simulink model "Sliders_mdl"  (R2018b)
settings: Solver=VariableStepAuto  StartTime=0.0  StopTime=10  MaxStep=0.01  RelTol=1e-3  EnableMultiTasking=on
libraries: lpvlibrary x2, cstblocks x1, simulink x1
settings Model: Creator=Fernando  LastModifiedBy=ferna
settings OptimizationCC: LifeSpan=inf
settings DebuggingCC: SFUnexpectedBacktrackingDiag=warning  SFNoUnconditionalDefaultTransitionDiag=warning
settings SFSimCC: SimUseLocalCustomCode=off
settings RTWCC: RTWUseLocalCustomCode=off
settings CodeAppCC: StateflowObjectComments=on
settings GRTTargetCC: TargetLangStandard=C89/C90 (ANSI)  GeneratePreprocessorConditionals=Disable all
settings ConfigComp: CovMetricSettings=dw  CovHtmlReporting=on  CovSaveCumulativeToWorkspaceVar=on  CovSaveSingleToWorkspaceVar=on  CovExternalEMLEnable=off

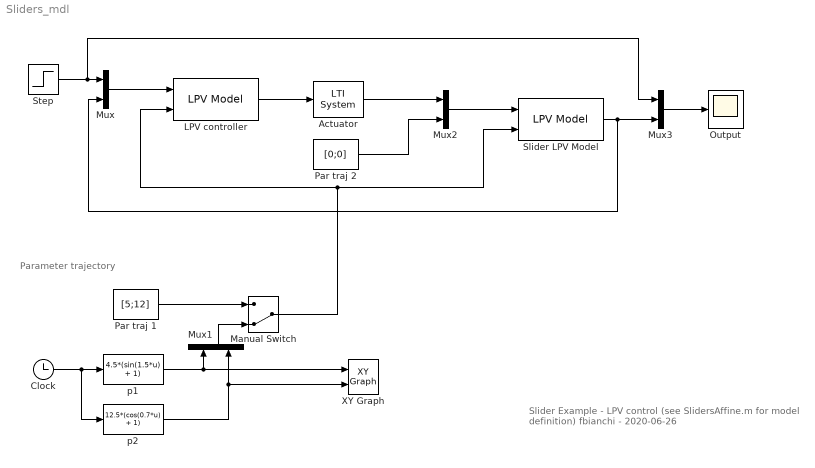
== system Sliders_mdl ==
  note: Slider Example - LPV control
      | (see SlidersAffine.m for model definition)
      | fbianchi - 2020-06-26
  note: Parameter trajectory
  Actuator : cstblocks/LTI System  sys=Act  IC=[]
  Clock : Clock
  LPV controller : lpvlibrary/LPV Model  pdSys=pdK1  x0=0
      settings: SourceProductName=LPV Toolbox
  Manual Switch : ManualSwitch  CurrentSetting=0
  Mux : Mux  Inputs=2
  Mux1 : Mux  Inputs=2
  Mux2 : Mux  Inputs=[1 2]
  Mux3 : Mux  Inputs=2
  Output : Scope
  Par traj 1 : Constant  Value=[5;12]
  Par traj 2 : Constant  Value=[0;0]
  Slider LPV Model : lpvlibrary/LPV Model  pdSys=pdG  x0=0
      settings: SourceProductName=LPV Toolbox
  Step : Step  Time=0.2  SampleTime=0
  XY Graph : simulink/Sinks/XY Graph  xmin=0  xmax=9  ymin=0  ymax=25  st=-1
  p1 : Fcn  Expr=4.5*(sin(1.5*u) + 1)
  p2 : Fcn  Expr=12.5*(cos(0.7*u) + 1)
  wires:
  Clock/1 -> p2/1, p1/1
  p1/1 -> XY Graph/1, Mux1/1
  p2/1 -> XY Graph/2, Mux1/2
  Mux1/1 -> Manual Switch/2
  Par traj 1/1 -> Manual Switch/1
  Step/1 -> Mux3/1, Mux/1
  Mux/1 -> LPV controller/1
  LPV controller/1 -> Actuator/1
  Actuator/1 -> Mux2/1
  Mux2/1 -> Slider LPV Model/1
  Par traj 2/1 -> Mux2/2
  Manual Switch/1 -> LPV controller/2, Slider LPV Model/2
  Slider LPV Model/1 -> Mux3/2, Mux/2
  Mux3/1 -> Output/1
